simulink model "GFLIB_Lut2D_BAM_FLT"  (Simulink 8.3)
settings: Solver=ode45  StartTime=0.0  StopTime=10.0  RelTol=1e-3
undefined symbols (not defined in the file): pfltTable, s32MidIdx, u32ShamOffset1, u32ShamOffset2
settings Model: Creator=B17364  LastModifiedBy=B17364
settings OptimizationCC: ExpressionDepthLimit=2147483647
settings DebuggingCC: FcnCallInpInsideContextMsg=UseLocalSettings  StrictBusMsg=Warning

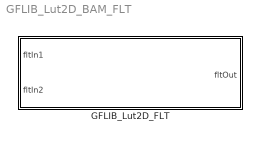
== system GFLIB_Lut2D_BAM_FLT ==
  GFLIB_Lut2D_FLT : Subsystem  mask(GFLIB_Lut2D_FLT){u32ShamOffset1=u32ShamOffset1, u32ShamOffset2=u32ShamOffset2, pfltTable=pfltTable, s32MidIdx=s32MidIdx}
      mask help: Bit accurate model of Lut2D function.
      mask init:
      | pos = get_param(gcb, 'Position');width = pos(3) - pos(1); height = pos(4) - pos(2);tX=width/2;tY=height*0.9;
      mask Display: color('black');port_label('input',1,'fltIn1');port_label('input',2,'fltIn2');port_label('output',1,'fltOut');color('black');disp('GFLIB_Lut2D_FLT');color('blue');text(tX,tY, 'BAM', 'horizontalAlignment', 'center');

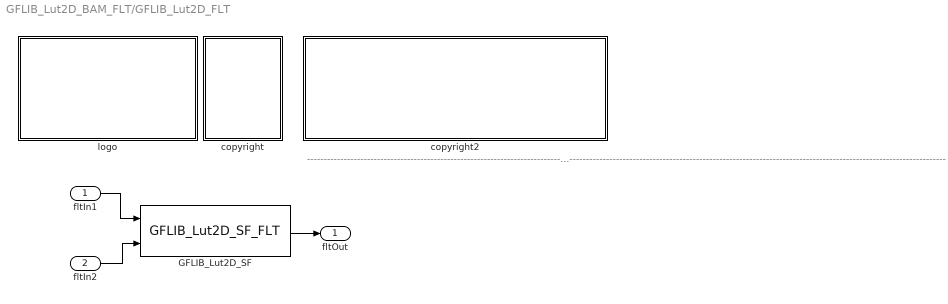
== system GFLIB_Lut2D_BAM_FLT/GFLIB_Lut2D_FLT ==
  note: ---------------------------------------------------------------------------------------------------------------------------------------------------------------------------------------------------
  fltIn1 : Inport
  fltIn2 : Inport  Port=2
  GFLIB_Lut2D_SF : S-Function  FunctionName=GFLIB_Lut2D_SF_FLT  Parameters=u32ShamOffset1,u32ShamOffset2,pfltTable,s32MidIdx  EnableBusSupport=off
  copyright : Subsystem
      mask Display:
      | text(10,90,'FILE:');text(10,75,'DESRIPTION:')
      | text(10,60,'COPYRIGHT:')
      | text(10,45,'VERSION:')
      | text(10,30,'DATE:')
  copyright2 : Subsystem
      mask Display:
      | text(10,90,'GFLIB_Lut2D_BAM_FLT.mdl');text(10,75,'Two dimensional Look-up table function');text(10,60,'Freescale')
      | text(10,45,'0.1');text(10,30,'17-Jun-2013');
  logo : Subsystem
      mask Display: image(imread('logo.jpg'))
  fltOut : Outport
  wires:
  fltIn1/1 -> GFLIB_Lut2D_SF/1
  fltIn2/1 -> GFLIB_Lut2D_SF/2
  GFLIB_Lut2D_SF/1 -> fltOut/1

== system GFLIB_Lut2D_BAM_FLT/GFLIB_Lut2D_FLT/copyright ==

== system GFLIB_Lut2D_BAM_FLT/GFLIB_Lut2D_FLT/copyright2 ==

== system GFLIB_Lut2D_BAM_FLT/GFLIB_Lut2D_FLT/logo ==
